simulink model "untitled"  (R2017b)
settings: Solver=VariableStepAuto  StartTime=0.0  StopTime=10.0  RelTol=1e-3
values from neighbouring files (symbols this model uses):
  d = 0.10    (= 0.1)    [main.m]
  kk = k/u*P1*P2    [main.m]
  P12 = -P1 -P2    [main.m]
  P1P2 = P1 * P2    [main.m]
  R = 0.056/2    (= 0.028)    [main.m]
libraries: simulink x3
settings Model: Creator=hoh  LastModifiedBy=Ale

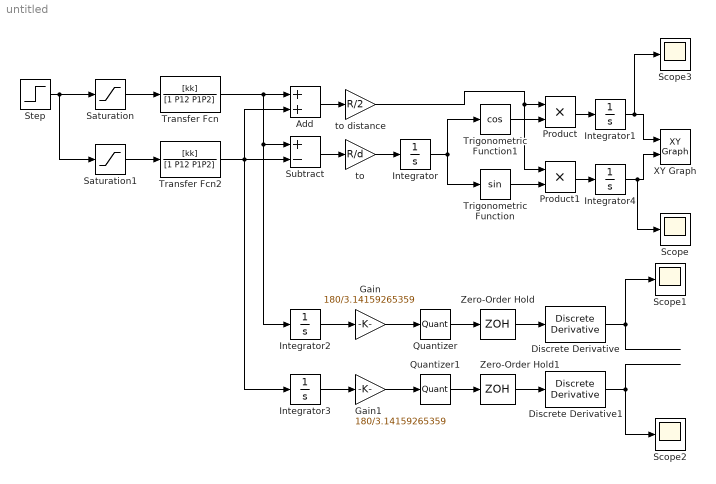
== system untitled ==
  Add : Sum
  Discrete Derivative : simulink/Discrete/Discrete Derivative  gainval=1  ICPrevScaledInput=0.0  OutMin=[]  OutMax=[]  OutDataType=fixdt(1, 16)  OutScaling=2^-10  DoSatur=off
  Discrete Derivative1 : simulink/Discrete/Discrete Derivative  gainval=1  ICPrevScaledInput=0.0  OutMin=[]  OutMax=[]  OutDataType=fixdt(1, 16)  OutScaling=2^-10  DoSatur=off
  Gain : Gain  Gain=180/3.14159265359
  Gain1 : Gain  Gain=180/3.14159265359
  Integrator{,1..4} (5 alike) : Integrator
  Product : Product
  Product1 : Product
  Quantizer : Quantizer  QuantizationInterval=1
  Quantizer1 : Quantizer  QuantizationInterval=1
  Saturation : Saturate  UpperLimit=100
  Saturation1 : Saturate  UpperLimit=100
  Scope{,1..3} (4 alike) : Scope
  Step : Step  Time=0  After=1000000  SampleTime=0
  Subtract : Sum  Inputs=+-
  Transfer Fcn : TransferFcn  Numerator=[kk]  Denominator=[1 P12 P1P2]
  Transfer Fcn2 : TransferFcn  Numerator=[kk]  Denominator=[1 P12 P1P2]
  Trigonometric Function : Trigonometry
  Trigonometric Function1 : Trigonometry  Operator=cos
  XY Graph : simulink/Sinks/XY Graph  xmin=-1  xmax=1  ymin=-1  ymax=1  st=-1
  Zero-Order Hold : ZeroOrderHold  SampleTime=0.005
  Zero-Order Hold1 : ZeroOrderHold  SampleTime=0.005
  "to " : Gain  Gain=R/d
  to distance : Gain  Gain=R/2
  wires:
  Subtract/1 -> "to "/1
  Integrator/1 -> Trigonometric Function/1, Trigonometric Function1/1
  to distance/1 -> Product1/1, Product/1
  Product/1 -> Integrator1/1
  Integrator1/1 -> Scope3/1, XY Graph/1
  Product1/1 -> Integrator4/1
  Add/1 -> to distance/1
  "to "/1 -> Integrator/1
  Integrator2/1 -> Gain/1
  Gain/1 -> Quantizer/1
  Quantizer/1 -> Zero-Order Hold/1
  Zero-Order Hold/1 -> Discrete Derivative/1
  Transfer Fcn/1 -> Subtract/1, Integrator2/1, Add/1
  Transfer Fcn2/1 -> Integrator3/1, Subtract/2, Add/2
  Discrete Derivative/1 -> Scope1/1
  Quantizer1/1 -> Zero-Order Hold1/1
  Gain1/1 -> Quantizer1/1
  Discrete Derivative1/1 -> Scope2/1
  Integrator3/1 -> Gain1/1
  Zero-Order Hold1/1 -> Discrete Derivative1/1
  Trigonometric Function1/1 -> Product/2
  Trigonometric Function/1 -> Product1/2
  Integrator4/1 -> Scope/1, XY Graph/2
  Saturation1/1 -> Transfer Fcn2/1
  Saturation/1 -> Transfer Fcn/1
  Step/1 -> Saturation1/1, Saturation/1
